simulink model "acmee3"  (R2018b)
settings: Solver=VariableStepAuto  StartTime=0.0  StopTime=10  RelTol=1e-3
values from neighbouring files (symbols this model uses):
  A = R_t - R_inv    [TP1_ROB.m]    (also in Untitled.m = [0 1 0 0 ; 0 0 -9 0 ; 0 0 0 1;-1 0 0 0]; exocmee.m = [0 1 2/3;-1 -2 1;0 -3 1]; q1 (1).m = [0 1 0 0;0 0 -9 0;0 0 0 1;-1 0 0 0])
  B = jacobian(dx,u)    [ACMEE1.m]    (also in TPACMEE1.m; Untitled.m = [0 ; 0 ; 0 ; 0.1]; Untitled3.m; exocmee.m = [1;2;3])
  C = jacobian(y,[x1,x2])    [ACMEE1.m]    (also in TP1RPI.m = Kp*((1+To*s)/(1+To*double(b)*s)); TP3RPI.m = Kp*(1+a*T1*s)*(1+T2*s)/((1+b*T2*s)*(1+T1*s)); TPACMEE1.m; Untitled.m = [1 0 0 0 ; 0 0 1 0])
  L = double(AP1)    [ACMEE1.m]    (also in TPACMEE1.m; Untitled.m = Kd'; exocmee.m = place(A',C',a2)'; simpson.m = (K1+2*K2+4*K3)*HX/3)
undefined symbols (not defined in the file or in its folder): K9
settings Model: Creator=GCBµ  LastModifiedBy=GCBµ

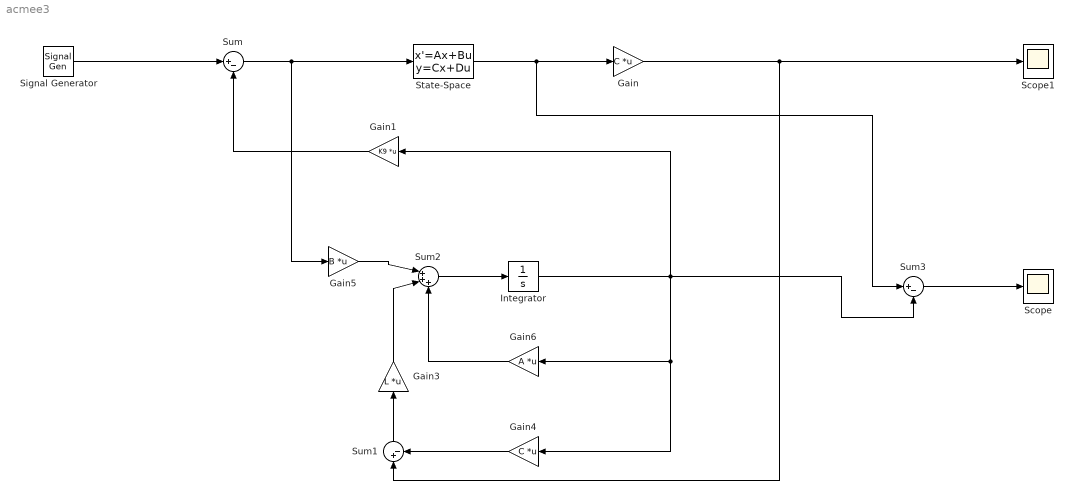
== system acmee3 ==
  Gain : Gain  Gain=C  Multiplication=Matrix(K*u)
  Gain1 : Gain  Gain=K9  Multiplication=Matrix(K*u)
  Gain3 : Gain  Gain=L  Multiplication=Matrix(K*u)
  Gain4 : Gain  Gain=C  Multiplication=Matrix(K*u)
  Gain5 : Gain  Gain=B  Multiplication=Matrix(K*u)
  Gain6 : Gain  Gain=A  Multiplication=Matrix(K*u)
  Integrator : Integrator
  Scope : Scope
  Scope1 : Scope
  Signal Generator : SignalGenerator
  State-Space : StateSpace  A=A  B=B  C=[1 0 0 0;0 1 0 0;0 0 1 0;0 0 0 1]  D=[0;0;0;0]  InitialCondition=[0.1;0;pi/12;0]
  Sum : Sum  Inputs=|+-
  Sum1 : Sum  Inputs=|+-
  Sum2 : Sum  Inputs=|+++
  Sum3 : Sum  Inputs=|+-
  wires:
  State-Space/1 -> Sum3/1, Gain/1
  Gain/1 -> Scope1/1, Sum1/1
  Sum/1 -> Gain5/1, State-Space/1
  Gain1/1 -> Sum/2
  Signal Generator/1 -> Sum/1
  Gain4/1 -> Sum1/2
  Gain6/1 -> Sum2/3
  Gain3/1 -> Sum2/2
  Sum1/1 -> Gain3/1
  Gain5/1 -> Sum2/1
  Sum2/1 -> Integrator/1
  Integrator/1 -> Sum3/2, Gain1/1, Gain6/1, Gain4/1
  Sum3/1 -> Scope/1
